simulink model "testbench_2"  (R2022b)
settings: Solver=VariableStepAuto  StartTime=0.0  StopTime=3600  RelTol=1e-3
undefined symbols (not defined in the file): battery_builder_rtmsupport, gcbh
libraries: nesl_utility x10, GD_Batterymodel_lib x8, fl_lib x2, BatteryCurrentManagement x1, BatteryBalancing x1
(part 1 of 2)
settings Model: Creator=DM  LastModifiedBy=DM

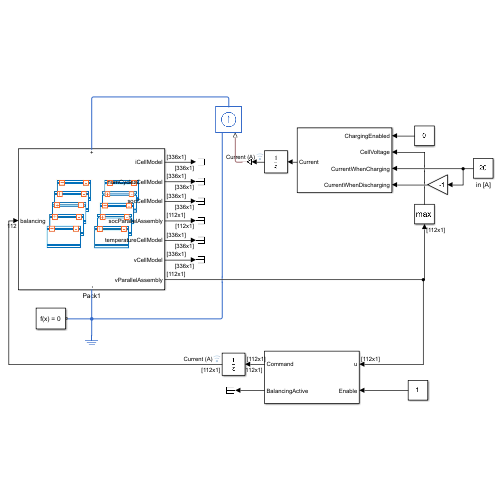
[thumbnail: Simulink's stored preview of the top-level diagram]
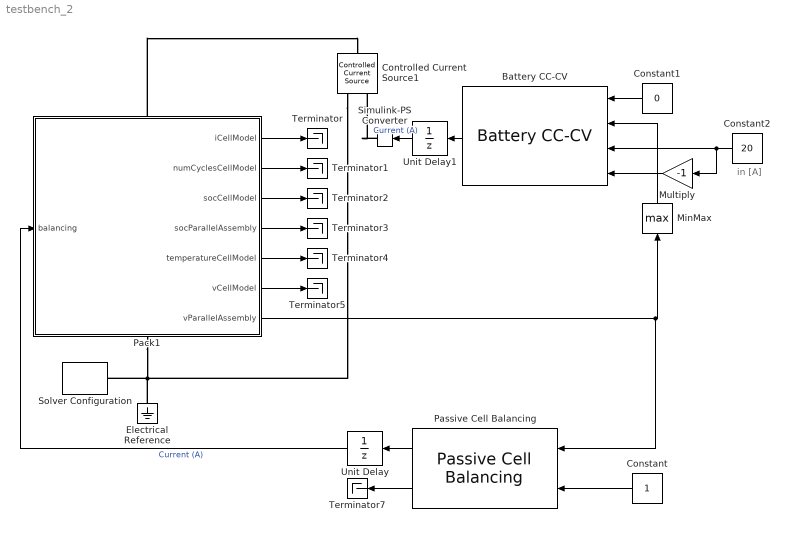
== system testbench_2 ==
  note: in [A]
  Battery CC-CV : BatteryCurrentManagement/Battery CC-CV  MaxCellVoltage=4.5  Kp=100  Ki=10  Kaw=1  Ts=-1
      settings: LibrarySourceBlock=batt_sl_lib/Current Management/Battery CC-CV
  Constant : Constant
  Constant1 : Constant  Value=0
  Constant2 : Constant  Value=20
  Controlled Current Source1 : fl_lib/Electrical/Electrical Sources/Controlled Current Source
  Electrical Reference : fl_lib/Electrical/Electrical Elements/Electrical Reference
  MinMax : MinMax  Function=max
  Multiply : Gain  Gain=-1
  Pack1 : Subsystem  LoadFcn=battery_builder_rtmsupport('loadfcn',gcbh);
      settings: CopyFcn=battery_builder_rtmsupport('copyfcn',gcbh);  PreCopyFcn=battery_builder_rtmsupport('precopyfcn',gcbh);  PreDeleteFcn=battery_builder_rtmsupport('predeletefcn',gcbh);  PortSchema="{\"entries\":[{\"content\":{\"sides\":[{\"content\":{\"connectorIds\":[\"LConn1\"]},\"type\":\"ConnectorPlacement.EquallySpacedRectSide\",\"uuid\":\"15f36c34-930d-4f52-9483-b00906672ad1\"},{\"content\":{\"connectorIds\":[\"RConn1\"],\"side\":\"RIGHT\"},\"type\":\"ConnectorPlacement.EquallySpacedRectSide\",\"uuid\":\"ac97c2df-2435-440c-95b5-222ce8189245\"},{\"content\":{\"connectorIds\":[\"In1\"],\"side\":\"TOP\"},\"type\":\"ConnectorPlacement.EquallySpacedRectSide\",\"uuid\":\"0c4398fe-7a4e-4114-b124-2a8e026b7d39\"},{\"content\":{\"connectorIds\":[\"Out1\",\"Out2\",\"Out3\",\"Out4\",\"Out5\",\"Out6\",\"Out7\"],\"side\":\"BOTTOM\"},\"type\":\"ConnectorPlacement.EquallySpacedRectSide\",\"uuid\":\"6740cf1b-9f23-4812-bda3-e18c05a0cb6c\"}]},\"type\":\"ConnectorPlacement.EquallySpacedConnector\",\"uuid\":\"12c02865-5fcb-4b07-b017-e8fa1f0f042b\"}],\"packageUris\":[\"http://schema.mathworks.com/mf0/Connector/R2020b\"],\"version\":\"1.0\"}"
      mask Display: image('$imagefile')
  Passive Cell Balancing : BatteryBalancing/Passive Cell Balancing  Threshold=0.2  Td_on=1  Td_off=1  Ts=-1
      settings: LibrarySourceBlock=batt_sl_lib/Cell Balancing/Passive Cell Balancing
  Simulink-PS Converter : nesl_utility/Simulink-PS Converter  PhysicalDomain=network_engine_domain  SubClassName=ps_input  LeftPortType=input  RightPortType=output  PseudoPeriodic=off  Frequencies=[]  NoiseDistribution=none  NoiseParameters=[]  Unit=1  AffineConversion=off  FilteringAndDerivatives=provide  SimscapeFilterOrder=1  InputFilterTimeConstant=0.001  UdotUserProvided=0
  Solver Configuration : nesl_utility/Solver Configuration  PhysicalDomain=network_engine_domain  SubClassName=solver  LeftPortType=input  RightPortType=generic  Tones=[]  Harmonics=[]  SimulateNoise=off  Profile=off  UseLocalSampling=off  EnableSwitchedLinearOptims=on  FrequencyDomain=off  UseCCode=off  RelTol=0.001  AbsTol=0.001  MinStep=1e-09  ToWorkspace=off  RevertToSquareIcSolve=off  NumHomotopyIterations=100  PhasorMode=off  PhasorModeNumHarmonics=1  ConsistencySolver=NEWTON_XTOL_AFTER_FTOL  IndexReductionMethod=DerivativeReplacement  DoDC=off  ResidualTolerance=1e-09  ConsistencyTolSource=GLOBAL  ConsistencyAbsTol=0.001  ConsistencyRelTol=0.001  ConsistencyTolFactor=0.001  UseLocalSolver=on  LocalSolverChoice=NE_BACKWARD_EULER_ADVANCER  ResolveIndetEquations=on  FunctionEvalNumThread=1  LocalSolverSampleTime=1  DoFixedCost=on  MaxNonlinIter=3  MaxModeIter=2  ComputeImpulses=off  ImpulseIterations=2  LinearAlgebra=auto  LinearAlgebraNumThread=0  EquationFormulation=NE_TIME_EF  DelaysMemoryBudget=1024  AutomaticFiltering=on  FilteringTimeConstant=0.001  PartitionStorageMethod=AS_NEEDED  PartitionMemoryBudget=1024  PartitionMethod=ROBUST
  Terminator{,1..5,7} (7 alike) : Terminator
  Unit Delay : UnitDelay  SampleTime=-1  HasFrameUpgradeWarning=on
  Unit Delay1 : UnitDelay  SampleTime=-1  HasFrameUpgradeWarning=on
  wires:
  Pack1/1(iCellModel) -> Terminator/1
  Pack1/2(numCyclesCellModel) -> Terminator1/1
  Pack1/3(socCellModel) -> Terminator2/1
  Pack1/4(socParallelAssembly) -> Terminator3/1
  Pack1/5(temperatureCellModel) -> Terminator4/1
  Pack1/6(vCellModel) -> Terminator5/1
  Passive Cell Balancing/2 -> Terminator7/1
  Constant/1 -> Passive Cell Balancing/2
  Constant1/1 -> Battery CC-CV/1
  Constant2/1 -> Multiply/1, Battery CC-CV/3
  Multiply/1 -> Battery CC-CV/4
  MinMax/1 -> Battery CC-CV/2
  Pack1/7(vParallelAssembly) -> Passive Cell Balancing/1, MinMax/1
  Passive Cell Balancing/1 -> Unit Delay/1
  Unit Delay/1 -> Pack1/1(balancing)  "Current (A)"
  Battery CC-CV/1 -> Unit Delay1/1
  Unit Delay1/1 -> Simulink-PS Converter/1  "Current (A)"
  connections:
  Pack1/LConn1 -- Controlled Current Source1/LConn1
  Electrical Reference/LConn1 -- Pack1/RConn1 -- Controlled Current Source1/RConn2 -- Solver Configuration/RConn1
  Simulink-PS Converter/RConn1 -- Controlled Current Source1/RConn1

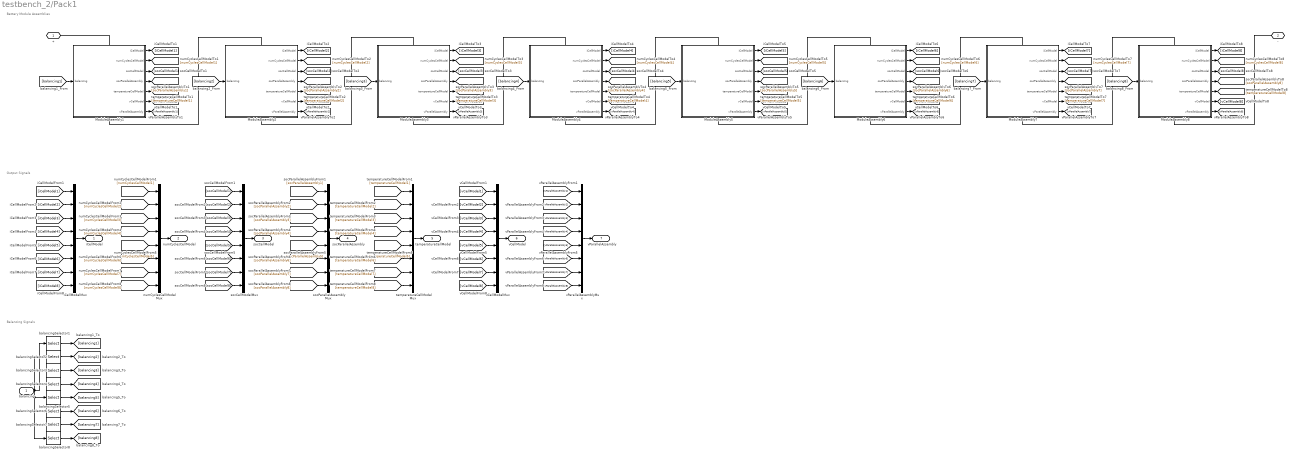
== system testbench_2/Pack1 ==
  note: Balancing Signals
  note: Output Signals
  note: Battery Module Assemblies
  balancing : Inport  PortDimensions=112
  ModuleAssembly1 : Subsystem  LoadFcn=battery_builder_rtmsupport('loadfcn',gcbh);
      settings: CopyFcn=battery_builder_rtmsupport('copyfcn',gcbh);  PreCopyFcn=battery_builder_rtmsupport('precopyfcn',gcbh);  PreDeleteFcn=battery_builder_rtmsupport('predeletefcn',gcbh);  PortSchema="{\"entries\":[{\"content\":{\"sides\":[{\"content\":{\"connectorIds\":[\"LConn1\"]},\"type\":\"ConnectorPlacement.EquallySpacedRectSide\",\"uuid\":\"15f36c34-930d-4f52-9483-b00906672ad1\"},{\"content\":{\"connectorIds\":[\"RConn1\"],\"side\":\"RIGHT\"},\"type\":\"ConnectorPlacement.EquallySpacedRectSide\",\"uuid\":\"ac97c2df-2435-440c-95b5-222ce8189245\"},{\"content\":{\"connectorIds\":[\"In1\"],\"side\":\"TOP\"},\"type\":\"ConnectorPlacement.EquallySpacedRectSide\",\"uuid\":\"0c4398fe-7a4e-4114-b124-2a8e026b7d39\"},{\"content\":{\"connectorIds\":[\"Out1\",\"Out2\",\"Out3\",\"Out4\",\"Out5\",\"Out6\",\"Out7\"],\"side\":\"BOTTOM\"},\"type\":\"ConnectorPlacement.EquallySpacedRectSide\",\"uuid\":\"5e29da8d-14fb-4ee5-a8e5-61c3c254e31c\"}]},\"type\":\"ConnectorPlacement.EquallySpacedConnector\",\"uuid\":\"12c02865-5fcb-4b07-b017-e8fa1f0f042b\"}],\"packageUris\":[\"http://schema.mathworks.com/mf0/Connector/R2020b\"],\"version\":\"1.0\"}"
      mask Display: image('$imagefile')
  ModuleAssembly2 : Subsystem  LoadFcn=battery_builder_rtmsupport('loadfcn',gcbh);
      settings: CopyFcn=battery_builder_rtmsupport('copyfcn',gcbh);  PreCopyFcn=battery_builder_rtmsupport('precopyfcn',gcbh);  PreDeleteFcn=battery_builder_rtmsupport('predeletefcn',gcbh);  PortSchema="{\"entries\":[{\"content\":{\"sides\":[{\"content\":{\"connectorIds\":[\"LConn1\"]},\"type\":\"ConnectorPlacement.EquallySpacedRectSide\",\"uuid\":\"15f36c34-930d-4f52-9483-b00906672ad1\"},{\"content\":{\"connectorIds\":[\"RConn1\"],\"side\":\"RIGHT\"},\"type\":\"ConnectorPlacement.EquallySpacedRectSide\",\"uuid\":\"ac97c2df-2435-440c-95b5-222ce8189245\"},{\"content\":{\"connectorIds\":[\"In1\"],\"side\":\"TOP\"},\"type\":\"ConnectorPlacement.EquallySpacedRectSide\",\"uuid\":\"0c4398fe-7a4e-4114-b124-2a8e026b7d39\"},{\"content\":{\"connectorIds\":[\"Out1\",\"Out2\",\"Out3\",\"Out4\",\"Out5\",\"Out6\",\"Out7\"],\"side\":\"BOTTOM\"},\"type\":\"ConnectorPlacement.EquallySpacedRectSide\",\"uuid\":\"5e29da8d-14fb-4ee5-a8e5-61c3c254e31c\"}]},\"type\":\"ConnectorPlacement.EquallySpacedConnector\",\"uuid\":\"12c02865-5fcb-4b07-b017-e8fa1f0f042b\"}],\"packageUris\":[\"http://schema.mathworks.com/mf0/Connector/R2020b\"],\"version\":\"1.0\"}"
      mask Display: image('$imagefile')
  ModuleAssembly3 : Subsystem  LoadFcn=battery_builder_rtmsupport('loadfcn',gcbh);
      settings: CopyFcn=battery_builder_rtmsupport('copyfcn',gcbh);  PreCopyFcn=battery_builder_rtmsupport('precopyfcn',gcbh);  PreDeleteFcn=battery_builder_rtmsupport('predeletefcn',gcbh);  PortSchema="{\"entries\":[{\"content\":{\"sides\":[{\"content\":{\"connectorIds\":[\"LConn1\"]},\"type\":\"ConnectorPlacement.EquallySpacedRectSide\",\"uuid\":\"15f36c34-930d-4f52-9483-b00906672ad1\"},{\"content\":{\"connectorIds\":[\"RConn1\"],\"side\":\"RIGHT\"},\"type\":\"ConnectorPlacement.EquallySpacedRectSide\",\"uuid\":\"ac97c2df-2435-440c-95b5-222ce8189245\"},{\"content\":{\"connectorIds\":[\"In1\"],\"side\":\"TOP\"},\"type\":\"ConnectorPlacement.EquallySpacedRectSide\",\"uuid\":\"0c4398fe-7a4e-4114-b124-2a8e026b7d39\"},{\"content\":{\"connectorIds\":[\"Out1\",\"Out2\",\"Out3\",\"Out4\",\"Out5\",\"Out6\",\"Out7\"],\"side\":\"BOTTOM\"},\"type\":\"ConnectorPlacement.EquallySpacedRectSide\",\"uuid\":\"5e29da8d-14fb-4ee5-a8e5-61c3c254e31c\"}]},\"type\":\"ConnectorPlacement.EquallySpacedConnector\",\"uuid\":\"12c02865-5fcb-4b07-b017-e8fa1f0f042b\"}],\"packageUris\":[\"http://schema.mathworks.com/mf0/Connector/R2020b\"],\"version\":\"1.0\"}"
      mask Display: image('$imagefile')
  ModuleAssembly4 : Subsystem  LoadFcn=battery_builder_rtmsupport('loadfcn',gcbh);
      settings: CopyFcn=battery_builder_rtmsupport('copyfcn',gcbh);  PreCopyFcn=battery_builder_rtmsupport('precopyfcn',gcbh);  PreDeleteFcn=battery_builder_rtmsupport('predeletefcn',gcbh);  PortSchema="{\"entries\":[{\"content\":{\"sides\":[{\"content\":{\"connectorIds\":[\"LConn1\"]},\"type\":\"ConnectorPlacement.EquallySpacedRectSide\",\"uuid\":\"15f36c34-930d-4f52-9483-b00906672ad1\"},{\"content\":{\"connectorIds\":[\"RConn1\"],\"side\":\"RIGHT\"},\"type\":\"ConnectorPlacement.EquallySpacedRectSide\",\"uuid\":\"ac97c2df-2435-440c-95b5-222ce8189245\"},{\"content\":{\"connectorIds\":[\"In1\"],\"side\":\"TOP\"},\"type\":\"ConnectorPlacement.EquallySpacedRectSide\",\"uuid\":\"0c4398fe-7a4e-4114-b124-2a8e026b7d39\"},{\"content\":{\"connectorIds\":[\"Out1\",\"Out2\",\"Out3\",\"Out4\",\"Out5\",\"Out6\",\"Out7\"],\"side\":\"BOTTOM\"},\"type\":\"ConnectorPlacement.EquallySpacedRectSide\",\"uuid\":\"5e29da8d-14fb-4ee5-a8e5-61c3c254e31c\"}]},\"type\":\"ConnectorPlacement.EquallySpacedConnector\",\"uuid\":\"12c02865-5fcb-4b07-b017-e8fa1f0f042b\"}],\"packageUris\":[\"http://schema.mathworks.com/mf0/Connector/R2020b\"],\"version\":\"1.0\"}"
      mask Display: image('$imagefile')
  ModuleAssembly5 : Subsystem  LoadFcn=battery_builder_rtmsupport('loadfcn',gcbh);
      settings: CopyFcn=battery_builder_rtmsupport('copyfcn',gcbh);  PreCopyFcn=battery_builder_rtmsupport('precopyfcn',gcbh);  PreDeleteFcn=battery_builder_rtmsupport('predeletefcn',gcbh);  PortSchema="{\"entries\":[{\"content\":{\"sides\":[{\"content\":{\"connectorIds\":[\"LConn1\"]},\"type\":\"ConnectorPlacement.EquallySpacedRectSide\",\"uuid\":\"15f36c34-930d-4f52-9483-b00906672ad1\"},{\"content\":{\"connectorIds\":[\"RConn1\"],\"side\":\"RIGHT\"},\"type\":\"ConnectorPlacement.EquallySpacedRectSide\",\"uuid\":\"ac97c2df-2435-440c-95b5-222ce8189245\"},{\"content\":{\"connectorIds\":[\"In1\"],\"side\":\"TOP\"},\"type\":\"ConnectorPlacement.EquallySpacedRectSide\",\"uuid\":\"0c4398fe-7a4e-4114-b124-2a8e026b7d39\"},{\"content\":{\"connectorIds\":[\"Out1\",\"Out2\",\"Out3\",\"Out4\",\"Out5\",\"Out6\",\"Out7\"],\"side\":\"BOTTOM\"},\"type\":\"ConnectorPlacement.EquallySpacedRectSide\",\"uuid\":\"5e29da8d-14fb-4ee5-a8e5-61c3c254e31c\"}]},\"type\":\"ConnectorPlacement.EquallySpacedConnector\",\"uuid\":\"12c02865-5fcb-4b07-b017-e8fa1f0f042b\"}],\"packageUris\":[\"http://schema.mathworks.com/mf0/Connector/R2020b\"],\"version\":\"1.0\"}"
      mask Display: image('$imagefile')
  ModuleAssembly6 : Subsystem  LoadFcn=battery_builder_rtmsupport('loadfcn',gcbh);
      settings: CopyFcn=battery_builder_rtmsupport('copyfcn',gcbh);  PreCopyFcn=battery_builder_rtmsupport('precopyfcn',gcbh);  PreDeleteFcn=battery_builder_rtmsupport('predeletefcn',gcbh);  PortSchema="{\"entries\":[{\"content\":{\"sides\":[{\"content\":{\"connectorIds\":[\"LConn1\"]},\"type\":\"ConnectorPlacement.EquallySpacedRectSide\",\"uuid\":\"15f36c34-930d-4f52-9483-b00906672ad1\"},{\"content\":{\"connectorIds\":[\"RConn1\"],\"side\":\"RIGHT\"},\"type\":\"ConnectorPlacement.EquallySpacedRectSide\",\"uuid\":\"ac97c2df-2435-440c-95b5-222ce8189245\"},{\"content\":{\"connectorIds\":[\"In1\"],\"side\":\"TOP\"},\"type\":\"ConnectorPlacement.EquallySpacedRectSide\",\"uuid\":\"0c4398fe-7a4e-4114-b124-2a8e026b7d39\"},{\"content\":{\"connectorIds\":[\"Out1\",\"Out2\",\"Out3\",\"Out4\",\"Out5\",\"Out6\",\"Out7\"],\"side\":\"BOTTOM\"},\"type\":\"ConnectorPlacement.EquallySpacedRectSide\",\"uuid\":\"5e29da8d-14fb-4ee5-a8e5-61c3c254e31c\"}]},\"type\":\"ConnectorPlacement.EquallySpacedConnector\",\"uuid\":\"12c02865-5fcb-4b07-b017-e8fa1f0f042b\"}],\"packageUris\":[\"http://schema.mathworks.com/mf0/Connector/R2020b\"],\"version\":\"1.0\"}"
      mask Display: image('$imagefile')
  ModuleAssembly7 : Subsystem  LoadFcn=battery_builder_rtmsupport('loadfcn',gcbh);
      settings: CopyFcn=battery_builder_rtmsupport('copyfcn',gcbh);  PreCopyFcn=battery_builder_rtmsupport('precopyfcn',gcbh);  PreDeleteFcn=battery_builder_rtmsupport('predeletefcn',gcbh);  PortSchema="{\"entries\":[{\"content\":{\"sides\":[{\"content\":{\"connectorIds\":[\"LConn1\"]},\"type\":\"ConnectorPlacement.EquallySpacedRectSide\",\"uuid\":\"15f36c34-930d-4f52-9483-b00906672ad1\"},{\"content\":{\"connectorIds\":[\"RConn1\"],\"side\":\"RIGHT\"},\"type\":\"ConnectorPlacement.EquallySpacedRectSide\",\"uuid\":\"ac97c2df-2435-440c-95b5-222ce8189245\"},{\"content\":{\"connectorIds\":[\"In1\"],\"side\":\"TOP\"},\"type\":\"ConnectorPlacement.EquallySpacedRectSide\",\"uuid\":\"0c4398fe-7a4e-4114-b124-2a8e026b7d39\"},{\"content\":{\"connectorIds\":[\"Out1\",\"Out2\",\"Out3\",\"Out4\",\"Out5\",\"Out6\",\"Out7\"],\"side\":\"BOTTOM\"},\"type\":\"ConnectorPlacement.EquallySpacedRectSide\",\"uuid\":\"5e29da8d-14fb-4ee5-a8e5-61c3c254e31c\"}]},\"type\":\"ConnectorPlacement.EquallySpacedConnector\",\"uuid\":\"12c02865-5fcb-4b07-b017-e8fa1f0f042b\"}],\"packageUris\":[\"http://schema.mathworks.com/mf0/Connector/R2020b\"],\"version\":\"1.0\"}"
      mask Display: image('$imagefile')
  ModuleAssembly8 : Subsystem  LoadFcn=battery_builder_rtmsupport('loadfcn',gcbh);
      settings: CopyFcn=battery_builder_rtmsupport('copyfcn',gcbh);  PreCopyFcn=battery_builder_rtmsupport('precopyfcn',gcbh);  PreDeleteFcn=battery_builder_rtmsupport('predeletefcn',gcbh);  PortSchema="{\"entries\":[{\"content\":{\"sides\":[{\"content\":{\"connectorIds\":[\"LConn1\"]},\"type\":\"ConnectorPlacement.EquallySpacedRectSide\",\"uuid\":\"15f36c34-930d-4f52-9483-b00906672ad1\"},{\"content\":{\"connectorIds\":[\"RConn1\"],\"side\":\"RIGHT\"},\"type\":\"ConnectorPlacement.EquallySpacedRectSide\",\"uuid\":\"ac97c2df-2435-440c-95b5-222ce8189245\"},{\"content\":{\"connectorIds\":[\"In1\"],\"side\":\"TOP\"},\"type\":\"ConnectorPlacement.EquallySpacedRectSide\",\"uuid\":\"0c4398fe-7a4e-4114-b124-2a8e026b7d39\"},{\"content\":{\"connectorIds\":[\"Out1\",\"Out2\",\"Out3\",\"Out4\",\"Out5\",\"Out6\",\"Out7\"],\"side\":\"BOTTOM\"},\"type\":\"ConnectorPlacement.EquallySpacedRectSide\",\"uuid\":\"5e29da8d-14fb-4ee5-a8e5-61c3c254e31c\"}]},\"type\":\"ConnectorPlacement.EquallySpacedConnector\",\"uuid\":\"12c02865-5fcb-4b07-b017-e8fa1f0f042b\"}],\"packageUris\":[\"http://schema.mathworks.com/mf0/Connector/R2020b\"],\"version\":\"1.0\"}"
      mask Display: image('$imagefile')
  balancingSelector1 : Selector  InputPortWidth=112  IndexOptions=Index vector (dialog)  Indices="[1   2   3   4   5   6   7   8   9  10  11  12  13  14]"  OutputSizes=1
  balancingSelector2 : Selector  InputPortWidth=112  IndexOptions=Index vector (dialog)  Indices="[15  16  17  18  19  20  21  22  23  24  25  26  27  28]"  OutputSizes=1
  balancingSelector3 : Selector  InputPortWidth=112  IndexOptions=Index vector (dialog)  Indices="[29  30  31  32  33  34  35  36  37  38  39  40  41  42]"  OutputSizes=1
  balancingSelector4 : Selector  InputPortWidth=112  IndexOptions=Index vector (dialog)  Indices="[43  44  45  46  47  48  49  50  51  52  53  54  55  56]"  OutputSizes=1
  balancingSelector5 : Selector  InputPortWidth=112  IndexOptions=Index vector (dialog)  Indices="[57  58  59  60  61  62  63  64  65  66  67  68  69  70]"  OutputSizes=1
  balancingSelector6 : Selector  InputPortWidth=112  IndexOptions=Index vector (dialog)  Indices="[71  72  73  74  75  76  77  78  79  80  81  82  83  84]"  OutputSizes=1
  balancingSelector7 : Selector  InputPortWidth=112  IndexOptions=Index vector (dialog)  Indices="[85  86  87  88  89  90  91  92  93  94  95  96  97  98]"  OutputSizes=1
  balancingSelector8 : Selector  InputPortWidth=112  IndexOptions=Index vector (dialog)  Indices="[99  100  101  102  103  104  105  106  107  108  109  110  111  112]"  OutputSizes=1
  iCellModelMux : Mux  Inputs=8
  numCyclesCellModelMux : Mux  Inputs=8
  socCellModelMux : Mux  Inputs=8
  socParallelAssemblyMux : Mux  Inputs=8
  temperatureCellModelMux : Mux  Inputs=8
  vCellModelMux : Mux  Inputs=8
  vParallelAssemblyMux : Mux  Inputs=8
  + : PMIOPort  Side=Left
  - : PMIOPort  Port=2  Side=Right
  iCellModel : Outport
  numCyclesCellModel : Outport  Port=2
  socCellModel : Outport  Port=3
  socParallelAssembly : Outport  Port=4
  temperatureCellModel : Outport  Port=5
  vCellModel : Outport  Port=6
  vParallelAssembly : Outport  Port=7
  wires:
  [balancing8] -> ModuleAssembly8/1(balancing)
  balancingSelector8/1 -> [balancing8]
  [balancing7] -> ModuleAssembly7/1(balancing)
  balancingSelector7/1 -> [balancing7]
  [balancing6] -> ModuleAssembly6/1(balancing)
  balancingSelector6/1 -> [balancing6]
  [balancing5] -> ModuleAssembly5/1(balancing)
  balancingSelector5/1 -> [balancing5]
  [balancing4] -> ModuleAssembly4/1(balancing)
  balancingSelector4/1 -> [balancing4]
  [balancing3] -> ModuleAssembly3/1(balancing)
  balancingSelector3/1 -> [balancing3]
  [balancing2] -> ModuleAssembly2/1(balancing)
  balancingSelector2/1 -> [balancing2]
  [balancing1] -> ModuleAssembly1/1(balancing)
  balancing/1 -> balancingSelector1/1, balancingSelector4/1, balancingSelector3/1, balancingSelector2/1, balancingSelector5/1, balancingSelector6/1, balancingSelector8/1, balancingSelector7/1
  balancingSelector1/1 -> [balancing1]
  [vParallelAssembly8] -> vParallelAssemblyMux/8
  ModuleAssembly8/7(vParallelAssembly) -> [vParallelAssembly8]
  [vCellModel8] -> vCellModelMux/8
  ModuleAssembly8/6(vCellModel) -> [vCellModel8]
  [temperatureCellModel8] -> temperatureCellModelMux/8
  ModuleAssembly8/5(temperatureCellModel) -> [temperatureCellModel8]
  [socParallelAssembly8] -> socParallelAssemblyMux/8
  ModuleAssembly8/4(socParallelAssembly) -> [socParallelAssembly8]
  [socCellModel8] -> socCellModelMux/8
  ModuleAssembly8/3(socCellModel) -> [socCellModel8]
  [numCyclesCellModel8] -> numCyclesCellModelMux/8
  ModuleAssembly8/2(numCyclesCellModel) -> [numCyclesCellModel8]
  [iCellModel8] -> iCellModelMux/8
  ModuleAssembly8/1(iCellModel) -> [iCellModel8]
  [vParallelAssembly7] -> vParallelAssemblyMux/7
  ModuleAssembly7/7(vParallelAssembly) -> [vParallelAssembly7]
  [vCellModel7] -> vCellModelMux/7
  ModuleAssembly7/6(vCellModel) -> [vCellModel7]
  [temperatureCellModel7] -> temperatureCellModelMux/7
  ModuleAssembly7/5(temperatureCellModel) -> [temperatureCellModel7]
  [socParallelAssembly7] -> socParallelAssemblyMux/7
  ModuleAssembly7/4(socParallelAssembly) -> [socParallelAssembly7]
  [socCellModel7] -> socCellModelMux/7
  ModuleAssembly7/3(socCellModel) -> [socCellModel7]
  [numCyclesCellModel7] -> numCyclesCellModelMux/7
  ModuleAssembly7/2(numCyclesCellModel) -> [numCyclesCellModel7]
  [iCellModel7] -> iCellModelMux/7
  ModuleAssembly7/1(iCellModel) -> [iCellModel7]
  [vParallelAssembly6] -> vParallelAssemblyMux/6
  ModuleAssembly6/7(vParallelAssembly) -> [vParallelAssembly6]
  [vCellModel6] -> vCellModelMux/6
  ModuleAssembly6/6(vCellModel) -> [vCellModel6]
  [temperatureCellModel6] -> temperatureCellModelMux/6
  ModuleAssembly6/5(temperatureCellModel) -> [temperatureCellModel6]
  [socParallelAssembly6] -> socParallelAssemblyMux/6
  ModuleAssembly6/4(socParallelAssembly) -> [socParallelAssembly6]
  [socCellModel6] -> socCellModelMux/6
  ModuleAssembly6/3(socCellModel) -> [socCellModel6]
  [numCyclesCellModel6] -> numCyclesCellModelMux/6
  ModuleAssembly6/2(numCyclesCellModel) -> [numCyclesCellModel6]
  [iCellModel6] -> iCellModelMux/6
  ModuleAssembly6/1(iCellModel) -> [iCellModel6]
  [vParallelAssembly5] -> vParallelAssemblyMux/5
  ModuleAssembly5/7(vParallelAssembly) -> [vParallelAssembly5]
  [vCellModel5] -> vCellModelMux/5
  ModuleAssembly5/6(vCellModel) -> [vCellModel5]
  [temperatureCellModel5] -> temperatureCellModelMux/5
  ModuleAssembly5/5(temperatureCellModel) -> [temperatureCellModel5]
  [socParallelAssembly5] -> socParallelAssemblyMux/5
  ModuleAssembly5/4(socParallelAssembly) -> [socParallelAssembly5]
  [socCellModel5] -> socCellModelMux/5
  ModuleAssembly5/3(socCellModel) -> [socCellModel5]
  [numCyclesCellModel5] -> numCyclesCellModelMux/5
  ModuleAssembly5/2(numCyclesCellModel) -> [numCyclesCellModel5]
  [iCellModel5] -> iCellModelMux/5
  ModuleAssembly5/1(iCellModel) -> [iCellModel5]
  [vParallelAssembly4] -> vParallelAssemblyMux/4
  ModuleAssembly4/7(vParallelAssembly) -> [vParallelAssembly4]
  [vCellModel4] -> vCellModelMux/4
  ModuleAssembly4/6(vCellModel) -> [vCellModel4]
  [temperatureCellModel4] -> temperatureCellModelMux/4
  ModuleAssembly4/5(temperatureCellModel) -> [temperatureCellModel4]
  [socParallelAssembly4] -> socParallelAssemblyMux/4
  ModuleAssembly4/4(socParallelAssembly) -> [socParallelAssembly4]
  [socCellModel4] -> socCellModelMux/4
  ModuleAssembly4/3(socCellModel) -> [socCellModel4]
  [numCyclesCellModel4] -> numCyclesCellModelMux/4
  ModuleAssembly4/2(numCyclesCellModel) -> [numCyclesCellModel4]
  [iCellModel4] -> iCellModelMux/4
  ModuleAssembly4/1(iCellModel) -> [iCellModel4]
  [vParallelAssembly3] -> vParallelAssemblyMux/3
  ModuleAssembly3/7(vParallelAssembly) -> [vParallelAssembly3]
  [vCellModel3] -> vCellModelMux/3
  ModuleAssembly3/6(vCellModel) -> [vCellModel3]
  [temperatureCellModel3] -> temperatureCellModelMux/3
  ModuleAssembly3/5(temperatureCellModel) -> [temperatureCellModel3]
  [socParallelAssembly3] -> socParallelAssemblyMux/3
  ModuleAssembly3/4(socParallelAssembly) -> [socParallelAssembly3]
  [socCellModel3] -> socCellModelMux/3
  ModuleAssembly3/3(socCellModel) -> [socCellModel3]
  [numCyclesCellModel3] -> numCyclesCellModelMux/3
  ModuleAssembly3/2(numCyclesCellModel) -> [numCyclesCellModel3]
  [iCellModel3] -> iCellModelMux/3
  ModuleAssembly3/1(iCellModel) -> [iCellModel3]
  [vParallelAssembly2] -> vParallelAssemblyMux/2
  ModuleAssembly2/7(vParallelAssembly) -> [vParallelAssembly2]
  [vCellModel2] -> vCellModelMux/2
  ModuleAssembly2/6(vCellModel) -> [vCellModel2]
  [temperatureCellModel2] -> temperatureCellModelMux/2
  ModuleAssembly2/5(temperatureCellModel) -> [temperatureCellModel2]
  [socParallelAssembly2] -> socParallelAssemblyMux/2
  ModuleAssembly2/4(socParallelAssembly) -> [socParallelAssembly2]
  [socCellModel2] -> socCellModelMux/2
  ModuleAssembly2/3(socCellModel) -> [socCellModel2]
  [numCyclesCellModel2] -> numCyclesCellModelMux/2
  ModuleAssembly2/2(numCyclesCellModel) -> [numCyclesCellModel2]
  [iCellModel2] -> iCellModelMux/2
  ModuleAssembly2/1(iCellModel) -> [iCellModel2]
  [vParallelAssembly1] -> vParallelAssemblyMux/1
  vParallelAssemblyMux/1 -> vParallelAssembly/1
  ModuleAssembly1/7(vParallelAssembly) -> [vParallelAssembly1]
  [vCellModel1] -> vCellModelMux/1
  vCellModelMux/1 -> vCellModel/1
  ModuleAssembly1/6(vCellModel) -> [vCellModel1]
  [temperatureCellModel1] -> temperatureCellModelMux/1
  temperatureCellModelMux/1 -> temperatureCellModel/1
  ModuleAssembly1/5(temperatureCellModel) -> [temperatureCellModel1]
  [socParallelAssembly1] -> socParallelAssemblyMux/1
  socParallelAssemblyMux/1 -> socParallelAssembly/1
  ModuleAssembly1/4(socParallelAssembly) -> [socParallelAssembly1]
  [socCellModel1] -> socCellModelMux/1
  socCellModelMux/1 -> socCellModel/1
  ModuleAssembly1/3(socCellModel) -> [socCellModel1]
  [numCyclesCellModel1] -> numCyclesCellModelMux/1
  numCyclesCellModelMux/1 -> numCyclesCellModel/1
  ModuleAssembly1/2(numCyclesCellModel) -> [numCyclesCellModel1]
  [iCellModel1] -> iCellModelMux/1
  iCellModelMux/1 -> iCellModel/1
  ModuleAssembly1/1(iCellModel) -> [iCellModel1]
  connections:
  ModuleAssembly8/RConn1 -- -/RConn1
  ModuleAssembly1/LConn1 -- +/RConn1
  ModuleAssembly8/LConn1 -- ModuleAssembly7/RConn1
  ModuleAssembly7/LConn1 -- ModuleAssembly6/RConn1
  ModuleAssembly6/LConn1 -- ModuleAssembly5/RConn1
  ModuleAssembly5/LConn1 -- ModuleAssembly4/RConn1
  ModuleAssembly4/LConn1 -- ModuleAssembly3/RConn1
  ModuleAssembly3/LConn1 -- ModuleAssembly2/RConn1
  ModuleAssembly2/LConn1 -- ModuleAssembly1/RConn1

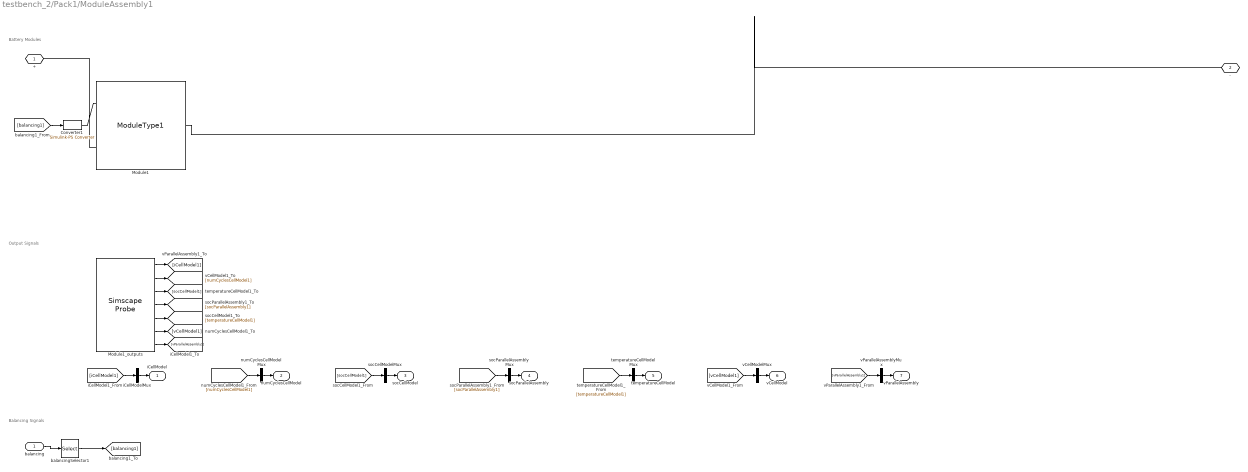
== system testbench_2/Pack1/ModuleAssembly1 ==
  note: Battery Modules
  note: Output Signals
  note: Balancing Signals
  balancing : Inport  PortDimensions=14
  Converter1 : nesl_utility/Simulink-PS Converter  PhysicalDomain=network_engine_domain  SubClassName=ps_input  LeftPortType=input  RightPortType=output  PseudoPeriodic=off  Frequencies=[]  NoiseDistribution=none  NoiseParameters=[]  Unit=1  AffineConversion=off  FilteringAndDerivatives=provide  SimscapeFilterOrder=1  InputFilterTimeConstant=0.001  UdotUserProvided=0
  Module1 : GD_Batterymodel_lib/Modules/ModuleType1  SOC_vec=[0, .1, .25, .5, .75, .9, 1]  T_vec=[278, 293, 313] K  V0_mat=[3.49, 3.5, 3.51; 3.55, 3.57, 3.56; 3.62, 3.63, 3.64; 3.71, 3.71, 3.72; 3.91, 3.93, 3.94; 4.07, 4.08, 4.08; 4.19, 4.19, 4.19] V  V_range=[0, inf] V  R0_mat=[.0117, .0085, .009; .011, .0085, .009; .0114, .0087, .0092; .0107, .0082, .0088; .0107, .0083, .0091; .0113, .0085, .0089; .0116, .0085, .0089] Ohm  AH=27 A*hr  extrapolation_option=simscape.enum.extrapolation.nearest  thermal_mass=100 J/K  CellBalancingClosedResistance=0.01 Ohm  CellBalancingOpenConductance=1e-8 1/Ohm  CellBalancingThreshold=0.5  CellBalancingResistance=50 Ohm  P=3  S=14  iCellModel_specify=off  iCellModel_priority=None  iCellModel=repmat(0, 42, 1) A  iCellModel_nominal_specify=off  iCellModel_nominal_unit=A  iCellModel_nominal_value=1  vCellModel_specify=off  vCellModel_priority=None  vCellModel=repmat(0, 42, 1) V  vCellModel_nominal_specify=off  vCellModel_nominal_unit=V  vCellModel_nominal_value=1  socCellModel_specify=off  socCellModel_priority=High  socCellModel=repmat(1, 42, 1)  socCellModel_nominal_specify=off  socCellModel_nominal_unit=1  socCellModel_nominal_value=1  numCyclesCellModel_specify=off  numCyclesCellModel_priority=High  numCyclesCellModel=repmat(0, 42, 1)  numCyclesCellModel_nominal_specify=off  numCyclesCellModel_nominal_unit=1  numCyclesCellModel_nominal_value=1  temperatureCellModel_specify=off  temperatureCellModel_priority=High  temperatureCellModel=repmat(298.15, 42, 1) K  temperatureCellModel_nominal_specify=off  temperatureCellModel_nominal_unit=K  temperatureCellModel_nominal_value=1  vParallelAssembly_specify=off  vParallelAssembly_priority=None  vParallelAssembly=repmat(0, 14, 1) V  vParallelAssembly_nominal_specify=off  vParallelAssembly_nominal_unit=V  vParallelAssembly_nominal_value=1  socParallelAssembly_specify=off  socParallelAssembly_priority=None  socParallelAssembly=repmat(1, 14, 1)  socParallelAssembly_nominal_specify=off  socParallelAssembly_nominal_unit=1  socParallelAssembly_nominal_value=1
      settings: InternalSimscapePortConfiguration="{\"Bottom\":[{\"id\":\"n\",\"label\":\"-\",\"type\":\"foundation.electrical.electrical\"}],\"Left\":[{\"id\":\"enableCellBalancing\",\"label\":\"CB\",\"type\":\"input\"}],\"Right\":[],\"Top\":[{\"id\":\"p\",\"label\":\"+\",\"type\":\"foundation.electrical.electrical\"}]}"
  Module1_outputs : SimscapeProbe  BoundBlock=522  Variables={iCellModel, numCyclesCellModel, socCellModel, socParallelAssembly, temperatureCellModel, vCellModel, vParallelAssembly}
  balancingSelector1 : Selector  InputPortWidth=14  IndexOptions=Index vector (dialog)  Indices="[1   2   3   4   5   6   7   8   9  10  11  12  13  14]"  OutputSizes=1
  iCellModelMux : Mux  Inputs=1
  numCyclesCellModelMux : Mux  Inputs=1
  socCellModelMux : Mux  Inputs=1
  socParallelAssemblyMux : Mux  Inputs=1
  temperatureCellModelMux : Mux  Inputs=1
  vCellModelMux : Mux  Inputs=1
  vParallelAssemblyMux : Mux  Inputs=1
  + : PMIOPort  Side=Left
  - : PMIOPort  Port=2  Side=Right
  iCellModel : Outport
  numCyclesCellModel : Outport  Port=2
  socCellModel : Outport  Port=3
  socParallelAssembly : Outport  Port=4
  temperatureCellModel : Outport  Port=5
  vCellModel : Outport  Port=6
  vParallelAssembly : Outport  Port=7
  wires:
  Module1_outputs/7 -> [vParallelAssembly1]
  iCellModelMux/1 -> iCellModel/1
  [iCellModel1] -> iCellModelMux/1
  Module1_outputs/6 -> [vCellModel1]
  numCyclesCellModelMux/1 -> numCyclesCellModel/1
  [numCyclesCellModel1] -> numCyclesCellModelMux/1
  Module1_outputs/5 -> [temperatureCellModel1]
  socCellModelMux/1 -> socCellModel/1
  [socCellModel1] -> socCellModelMux/1
  Module1_outputs/4 -> [socParallelAssembly1]
  socParallelAssemblyMux/1 -> socParallelAssembly/1
  [socParallelAssembly1] -> socParallelAssemblyMux/1
  Module1_outputs/3 -> [socCellModel1]
  temperatureCellModelMux/1 -> temperatureCellModel/1
  [temperatureCellModel1] -> temperatureCellModelMux/1
  Module1_outputs/2 -> [numCyclesCellModel1]
  vCellModelMux/1 -> vCellModel/1
  [vCellModel1] -> vCellModelMux/1
  Module1_outputs/1 -> [iCellModel1]
  vParallelAssemblyMux/1 -> vParallelAssembly/1
  [vParallelAssembly1] -> vParallelAssemblyMux/1
  balancing/1 -> balancingSelector1/1
  balancingSelector1/1 -> [balancing1]
  [balancing1] -> Converter1/1
  connections:
  Module1/LConn2 -- +/RConn1
  Module1/RConn1 -- -/RConn1
  Converter1/RConn1 -- Module1/LConn1

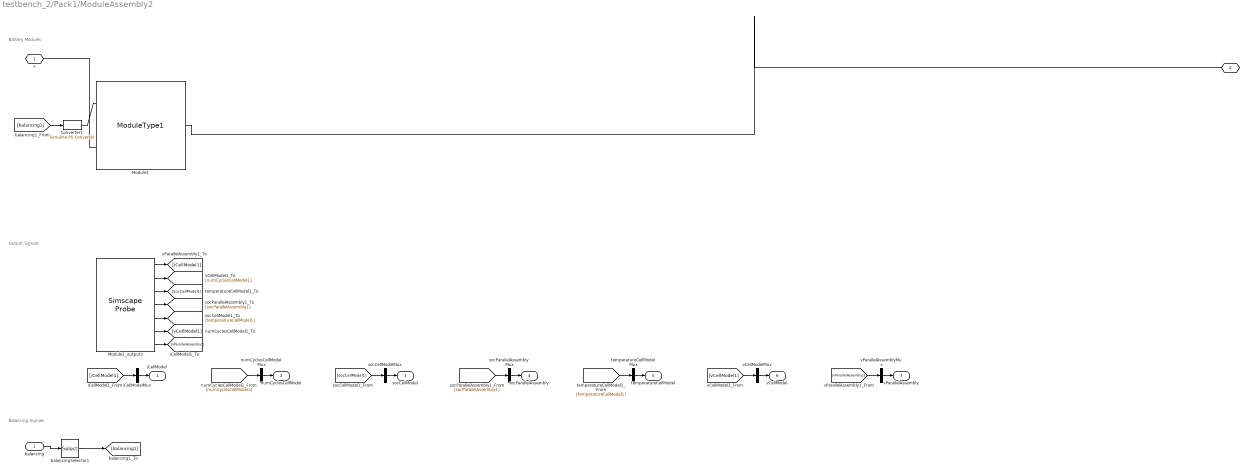
== system testbench_2/Pack1/ModuleAssembly2 ==
  note: Battery Modules
  note: Output Signals
  note: Balancing Signals
  balancing : Inport  PortDimensions=14
  Converter1 : nesl_utility/Simulink-PS Converter  PhysicalDomain=network_engine_domain  SubClassName=ps_input  LeftPortType=input  RightPortType=output  PseudoPeriodic=off  Frequencies=[]  NoiseDistribution=none  NoiseParameters=[]  Unit=1  AffineConversion=off  FilteringAndDerivatives=provide  SimscapeFilterOrder=1  InputFilterTimeConstant=0.001  UdotUserProvided=0
  Module1 : GD_Batterymodel_lib/Modules/ModuleType1  SOC_vec=[0, .1, .25, .5, .75, .9, 1]  T_vec=[278, 293, 313] K  V0_mat=[3.49, 3.5, 3.51; 3.55, 3.57, 3.56; 3.62, 3.63, 3.64; 3.71, 3.71, 3.72; 3.91, 3.93, 3.94; 4.07, 4.08, 4.08; 4.19, 4.19, 4.19] V  V_range=[0, inf] V  R0_mat=[.0117, .0085, .009; .011, .0085, .009; .0114, .0087, .0092; .0107, .0082, .0088; .0107, .0083, .0091; .0113, .0085, .0089; .0116, .0085, .0089] Ohm  AH=27 A*hr  extrapolation_option=simscape.enum.extrapolation.nearest  thermal_mass=100 J/K  CellBalancingClosedResistance=0.01 Ohm  CellBalancingOpenConductance=1e-8 1/Ohm  CellBalancingThreshold=0.5  CellBalancingResistance=50 Ohm  P=3  S=14  iCellModel_specify=off  iCellModel_priority=None  iCellModel=repmat(0, 42, 1) A  iCellModel_nominal_specify=off  iCellModel_nominal_unit=A  iCellModel_nominal_value=1  vCellModel_specify=off  vCellModel_priority=None  vCellModel=repmat(0, 42, 1) V  vCellModel_nominal_specify=off  vCellModel_nominal_unit=V  vCellModel_nominal_value=1  socCellModel_specify=off  socCellModel_priority=High  socCellModel=repmat(1, 42, 1)  socCellModel_nominal_specify=off  socCellModel_nominal_unit=1  socCellModel_nominal_value=1  numCyclesCellModel_specify=off  numCyclesCellModel_priority=High  numCyclesCellModel=repmat(0, 42, 1)  numCyclesCellModel_nominal_specify=off  numCyclesCellModel_nominal_unit=1  numCyclesCellModel_nominal_value=1  temperatureCellModel_specify=off  temperatureCellModel_priority=High  temperatureCellModel=repmat(298.15, 42, 1) K  temperatureCellModel_nominal_specify=off  temperatureCellModel_nominal_unit=K  temperatureCellModel_nominal_value=1  vParallelAssembly_specify=off  vParallelAssembly_priority=None  vParallelAssembly=repmat(0, 14, 1) V  vParallelAssembly_nominal_specify=off  vParallelAssembly_nominal_unit=V  vParallelAssembly_nominal_value=1  socParallelAssembly_specify=off  socParallelAssembly_priority=None  socParallelAssembly=repmat(1, 14, 1)  socParallelAssembly_nominal_specify=off  socParallelAssembly_nominal_unit=1  socParallelAssembly_nominal_value=1
      settings: InternalSimscapePortConfiguration="{\"Bottom\":[{\"id\":\"n\",\"label\":\"-\",\"type\":\"foundation.electrical.electrical\"}],\"Left\":[{\"id\":\"enableCellBalancing\",\"label\":\"CB\",\"type\":\"input\"}],\"Right\":[],\"Top\":[{\"id\":\"p\",\"label\":\"+\",\"type\":\"foundation.electrical.electrical\"}]}"
  Module1_outputs : SimscapeProbe  BoundBlock=563  Variables={iCellModel, numCyclesCellModel, socCellModel, socParallelAssembly, temperatureCellModel, vCellModel, vParallelAssembly}
  balancingSelector1 : Selector  InputPortWidth=14  IndexOptions=Index vector (dialog)  Indices="[1   2   3   4   5   6   7   8   9  10  11  12  13  14]"  OutputSizes=1
  iCellModelMux : Mux  Inputs=1
  numCyclesCellModelMux : Mux  Inputs=1
  socCellModelMux : Mux  Inputs=1
  socParallelAssemblyMux : Mux  Inputs=1
  temperatureCellModelMux : Mux  Inputs=1
  vCellModelMux : Mux  Inputs=1
  vParallelAssemblyMux : Mux  Inputs=1
  + : PMIOPort  Side=Left
  - : PMIOPort  Port=2  Side=Right
  iCellModel : Outport
  numCyclesCellModel : Outport  Port=2
  socCellModel : Outport  Port=3
  socParallelAssembly : Outport  Port=4
  temperatureCellModel : Outport  Port=5
  vCellModel : Outport  Port=6
  vParallelAssembly : Outport  Port=7
  wires:
  Module1_outputs/7 -> [vParallelAssembly1]
  iCellModelMux/1 -> iCellModel/1
  [iCellModel1] -> iCellModelMux/1
  Module1_outputs/6 -> [vCellModel1]
  numCyclesCellModelMux/1 -> numCyclesCellModel/1
  [numCyclesCellModel1] -> numCyclesCellModelMux/1
  Module1_outputs/5 -> [temperatureCellModel1]
  socCellModelMux/1 -> socCellModel/1
  [socCellModel1] -> socCellModelMux/1
  Module1_outputs/4 -> [socParallelAssembly1]
  socParallelAssemblyMux/1 -> socParallelAssembly/1
  [socParallelAssembly1] -> socParallelAssemblyMux/1
  Module1_outputs/3 -> [socCellModel1]
  temperatureCellModelMux/1 -> temperatureCellModel/1
  [temperatureCellModel1] -> temperatureCellModelMux/1
  Module1_outputs/2 -> [numCyclesCellModel1]
  vCellModelMux/1 -> vCellModel/1
  [vCellModel1] -> vCellModelMux/1
  Module1_outputs/1 -> [iCellModel1]
  vParallelAssemblyMux/1 -> vParallelAssembly/1
  [vParallelAssembly1] -> vParallelAssemblyMux/1
  balancing/1 -> balancingSelector1/1
  balancingSelector1/1 -> [balancing1]
  [balancing1] -> Converter1/1
  connections:
  Module1/LConn2 -- +/RConn1
  Module1/RConn1 -- -/RConn1
  Converter1/RConn1 -- Module1/LConn1

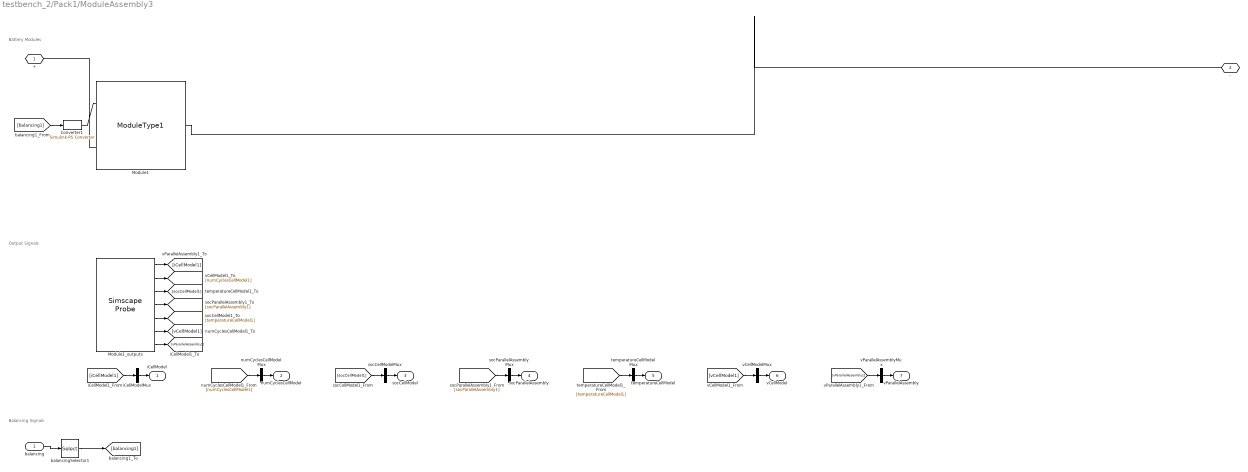
== system testbench_2/Pack1/ModuleAssembly3 ==
  note: Battery Modules
  note: Output Signals
  note: Balancing Signals
  balancing : Inport  PortDimensions=14
  Converter1 : nesl_utility/Simulink-PS Converter  PhysicalDomain=network_engine_domain  SubClassName=ps_input  LeftPortType=input  RightPortType=output  PseudoPeriodic=off  Frequencies=[]  NoiseDistribution=none  NoiseParameters=[]  Unit=1  AffineConversion=off  FilteringAndDerivatives=provide  SimscapeFilterOrder=1  InputFilterTimeConstant=0.001  UdotUserProvided=0
  Module1 : GD_Batterymodel_lib/Modules/ModuleType1  SOC_vec=[0, .1, .25, .5, .75, .9, 1]  T_vec=[278, 293, 313] K  V0_mat=[3.49, 3.5, 3.51; 3.55, 3.57, 3.56; 3.62, 3.63, 3.64; 3.71, 3.71, 3.72; 3.91, 3.93, 3.94; 4.07, 4.08, 4.08; 4.19, 4.19, 4.19] V  V_range=[0, inf] V  R0_mat=[.0117, .0085, .009; .011, .0085, .009; .0114, .0087, .0092; .0107, .0082, .0088; .0107, .0083, .0091; .0113, .0085, .0089; .0116, .0085, .0089] Ohm  AH=27 A*hr  extrapolation_option=simscape.enum.extrapolation.nearest  thermal_mass=100 J/K  CellBalancingClosedResistance=0.01 Ohm  CellBalancingOpenConductance=1e-8 1/Ohm  CellBalancingThreshold=0.5  CellBalancingResistance=50 Ohm  P=3  S=14  iCellModel_specify=off  iCellModel_priority=None  iCellModel=repmat(0, 42, 1) A  iCellModel_nominal_specify=off  iCellModel_nominal_unit=A  iCellModel_nominal_value=1  vCellModel_specify=off  vCellModel_priority=None  vCellModel=repmat(0, 42, 1) V  vCellModel_nominal_specify=off  vCellModel_nominal_unit=V  vCellModel_nominal_value=1  socCellModel_specify=off  socCellModel_priority=High  socCellModel=repmat(1, 42, 1)  socCellModel_nominal_specify=off  socCellModel_nominal_unit=1  socCellModel_nominal_value=1  numCyclesCellModel_specify=off  numCyclesCellModel_priority=High  numCyclesCellModel=repmat(0, 42, 1)  numCyclesCellModel_nominal_specify=off  numCyclesCellModel_nominal_unit=1  numCyclesCellModel_nominal_value=1  temperatureCellModel_specify=off  temperatureCellModel_priority=High  temperatureCellModel=repmat(298.15, 42, 1) K  temperatureCellModel_nominal_specify=off  temperatureCellModel_nominal_unit=K  temperatureCellModel_nominal_value=1  vParallelAssembly_specify=off  vParallelAssembly_priority=None  vParallelAssembly=repmat(0, 14, 1) V  vParallelAssembly_nominal_specify=off  vParallelAssembly_nominal_unit=V  vParallelAssembly_nominal_value=1  socParallelAssembly_specify=off  socParallelAssembly_priority=None  socParallelAssembly=repmat(1, 14, 1)  socParallelAssembly_nominal_specify=off  socParallelAssembly_nominal_unit=1  socParallelAssembly_nominal_value=1
      settings: InternalSimscapePortConfiguration="{\"Bottom\":[{\"id\":\"n\",\"label\":\"-\",\"type\":\"foundation.electrical.electrical\"}],\"Left\":[{\"id\":\"enableCellBalancing\",\"label\":\"CB\",\"type\":\"input\"}],\"Right\":[],\"Top\":[{\"id\":\"p\",\"label\":\"+\",\"type\":\"foundation.electrical.electrical\"}]}"
  Module1_outputs : SimscapeProbe  BoundBlock=604  Variables={iCellModel, numCyclesCellModel, socCellModel, socParallelAssembly, temperatureCellModel, vCellModel, vParallelAssembly}
  balancingSelector1 : Selector  InputPortWidth=14  IndexOptions=Index vector (dialog)  Indices="[1   2   3   4   5   6   7   8   9  10  11  12  13  14]"  OutputSizes=1
  iCellModelMux : Mux  Inputs=1
  numCyclesCellModelMux : Mux  Inputs=1
  socCellModelMux : Mux  Inputs=1
  socParallelAssemblyMux : Mux  Inputs=1
  temperatureCellModelMux : Mux  Inputs=1
  vCellModelMux : Mux  Inputs=1
  vParallelAssemblyMux : Mux  Inputs=1
  + : PMIOPort  Side=Left
  - : PMIOPort  Port=2  Side=Right
  iCellModel : Outport
  numCyclesCellModel : Outport  Port=2
  socCellModel : Outport  Port=3
  socParallelAssembly : Outport  Port=4
  temperatureCellModel : Outport  Port=5
  vCellModel : Outport  Port=6
  vParallelAssembly : Outport  Port=7
  wires:
  Module1_outputs/7 -> [vParallelAssembly1]
  iCellModelMux/1 -> iCellModel/1
  [iCellModel1] -> iCellModelMux/1
  Module1_outputs/6 -> [vCellModel1]
  numCyclesCellModelMux/1 -> numCyclesCellModel/1
  [numCyclesCellModel1] -> numCyclesCellModelMux/1
  Module1_outputs/5 -> [temperatureCellModel1]
  socCellModelMux/1 -> socCellModel/1
  [socCellModel1] -> socCellModelMux/1
  Module1_outputs/4 -> [socParallelAssembly1]
  socParallelAssemblyMux/1 -> socParallelAssembly/1
  [socParallelAssembly1] -> socParallelAssemblyMux/1
  Module1_outputs/3 -> [socCellModel1]
  temperatureCellModelMux/1 -> temperatureCellModel/1
  [temperatureCellModel1] -> temperatureCellModelMux/1
  Module1_outputs/2 -> [numCyclesCellModel1]
  vCellModelMux/1 -> vCellModel/1
  [vCellModel1] -> vCellModelMux/1
  Module1_outputs/1 -> [iCellModel1]
  vParallelAssemblyMux/1 -> vParallelAssembly/1
  [vParallelAssembly1] -> vParallelAssemblyMux/1
  balancing/1 -> balancingSelector1/1
  balancingSelector1/1 -> [balancing1]
  [balancing1] -> Converter1/1
  connections:
  Module1/LConn2 -- +/RConn1
  Module1/RConn1 -- -/RConn1
  Converter1/RConn1 -- Module1/LConn1

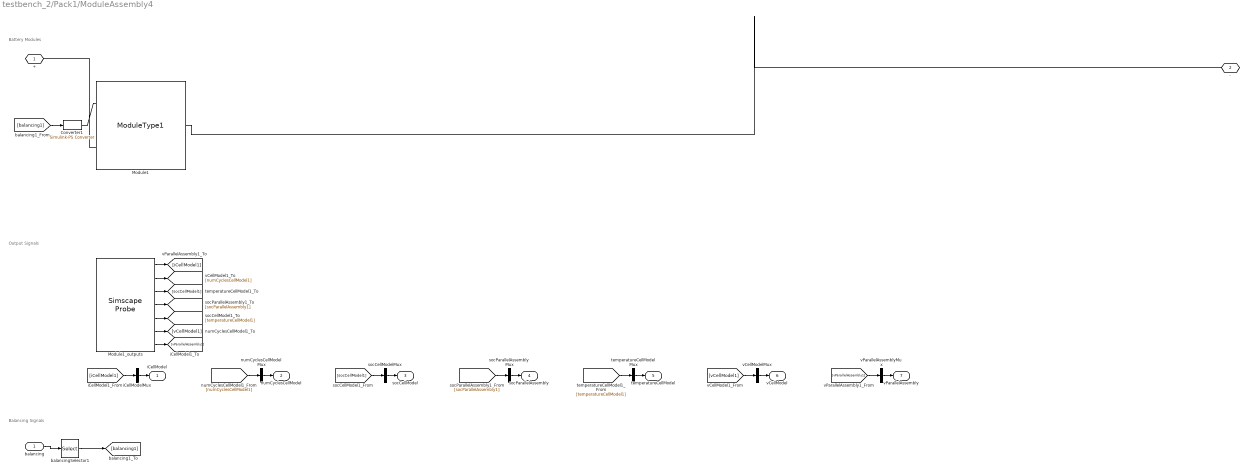
== system testbench_2/Pack1/ModuleAssembly4 ==
  note: Battery Modules
  note: Output Signals
  note: Balancing Signals
  balancing : Inport  PortDimensions=14
  Converter1 : nesl_utility/Simulink-PS Converter  PhysicalDomain=network_engine_domain  SubClassName=ps_input  LeftPortType=input  RightPortType=output  PseudoPeriodic=off  Frequencies=[]  NoiseDistribution=none  NoiseParameters=[]  Unit=1  AffineConversion=off  FilteringAndDerivatives=provide  SimscapeFilterOrder=1  InputFilterTimeConstant=0.001  UdotUserProvided=0
  Module1 : GD_Batterymodel_lib/Modules/ModuleType1  SOC_vec=[0, .1, .25, .5, .75, .9, 1]  T_vec=[278, 293, 313] K  V0_mat=[3.49, 3.5, 3.51; 3.55, 3.57, 3.56; 3.62, 3.63, 3.64; 3.71, 3.71, 3.72; 3.91, 3.93, 3.94; 4.07, 4.08, 4.08; 4.19, 4.19, 4.19] V  V_range=[0, inf] V  R0_mat=[.0117, .0085, .009; .011, .0085, .009; .0114, .0087, .0092; .0107, .0082, .0088; .0107, .0083, .0091; .0113, .0085, .0089; .0116, .0085, .0089] Ohm  AH=27 A*hr  extrapolation_option=simscape.enum.extrapolation.nearest  thermal_mass=100 J/K  CellBalancingClosedResistance=0.01 Ohm  CellBalancingOpenConductance=1e-8 1/Ohm  CellBalancingThreshold=0.5  CellBalancingResistance=50 Ohm  P=3  S=14  iCellModel_specify=off  iCellModel_priority=None  iCellModel=repmat(0, 42, 1) A  iCellModel_nominal_specify=off  iCellModel_nominal_unit=A  iCellModel_nominal_value=1  vCellModel_specify=off  vCellModel_priority=None  vCellModel=repmat(0, 42, 1) V  vCellModel_nominal_specify=off  vCellModel_nominal_unit=V  vCellModel_nominal_value=1  socCellModel_specify=off  socCellModel_priority=High  socCellModel=repmat(1, 42, 1)  socCellModel_nominal_specify=off  socCellModel_nominal_unit=1  socCellModel_nominal_value=1  numCyclesCellModel_specify=off  numCyclesCellModel_priority=High  numCyclesCellModel=repmat(0, 42, 1)  numCyclesCellModel_nominal_specify=off  numCyclesCellModel_nominal_unit=1  numCyclesCellModel_nominal_value=1  temperatureCellModel_specify=off  temperatureCellModel_priority=High  temperatureCellModel=repmat(298.15, 42, 1) K  temperatureCellModel_nominal_specify=off  temperatureCellModel_nominal_unit=K  temperatureCellModel_nominal_value=1  vParallelAssembly_specify=off  vParallelAssembly_priority=None  vParallelAssembly=repmat(0, 14, 1) V  vParallelAssembly_nominal_specify=off  vParallelAssembly_nominal_unit=V  vParallelAssembly_nominal_value=1  socParallelAssembly_specify=off  socParallelAssembly_priority=None  socParallelAssembly=repmat(1, 14, 1)  socParallelAssembly_nominal_specify=off  socParallelAssembly_nominal_unit=1  socParallelAssembly_nominal_value=1
      settings: InternalSimscapePortConfiguration="{\"Bottom\":[{\"id\":\"n\",\"label\":\"-\",\"type\":\"foundation.electrical.electrical\"}],\"Left\":[{\"id\":\"enableCellBalancing\",\"label\":\"CB\",\"type\":\"input\"}],\"Right\":[],\"Top\":[{\"id\":\"p\",\"label\":\"+\",\"type\":\"foundation.electrical.electrical\"}]}"
  Module1_outputs : SimscapeProbe  BoundBlock=645  Variables={iCellModel, numCyclesCellModel, socCellModel, socParallelAssembly, temperatureCellModel, vCellModel, vParallelAssembly}
  balancingSelector1 : Selector  InputPortWidth=14  IndexOptions=Index vector (dialog)  Indices="[1   2   3   4   5   6   7   8   9  10  11  12  13  14]"  OutputSizes=1
  iCellModelMux : Mux  Inputs=1
  numCyclesCellModelMux : Mux  Inputs=1
  socCellModelMux : Mux  Inputs=1
  socParallelAssemblyMux : Mux  Inputs=1
  temperatureCellModelMux : Mux  Inputs=1
  vCellModelMux : Mux  Inputs=1
  vParallelAssemblyMux : Mux  Inputs=1
  + : PMIOPort  Side=Left
  - : PMIOPort  Port=2  Side=Right
  iCellModel : Outport
  numCyclesCellModel : Outport  Port=2
  socCellModel : Outport  Port=3
  socParallelAssembly : Outport  Port=4
  temperatureCellModel : Outport  Port=5
  vCellModel : Outport  Port=6
  vParallelAssembly : Outport  Port=7
  wires:
  Module1_outputs/7 -> [vParallelAssembly1]
  iCellModelMux/1 -> iCellModel/1
  [iCellModel1] -> iCellModelMux/1
  Module1_outputs/6 -> [vCellModel1]
  numCyclesCellModelMux/1 -> numCyclesCellModel/1
  [numCyclesCellModel1] -> numCyclesCellModelMux/1
  Module1_outputs/5 -> [temperatureCellModel1]
  socCellModelMux/1 -> socCellModel/1
  [socCellModel1] -> socCellModelMux/1
  Module1_outputs/4 -> [socParallelAssembly1]
  socParallelAssemblyMux/1 -> socParallelAssembly/1
  [socParallelAssembly1] -> socParallelAssemblyMux/1
  Module1_outputs/3 -> [socCellModel1]
  temperatureCellModelMux/1 -> temperatureCellModel/1
  [temperatureCellModel1] -> temperatureCellModelMux/1
  Module1_outputs/2 -> [numCyclesCellModel1]
  vCellModelMux/1 -> vCellModel/1
  [vCellModel1] -> vCellModelMux/1
  Module1_outputs/1 -> [iCellModel1]
  vParallelAssemblyMux/1 -> vParallelAssembly/1
  [vParallelAssembly1] -> vParallelAssemblyMux/1
  balancing/1 -> balancingSelector1/1
  balancingSelector1/1 -> [balancing1]
  [balancing1] -> Converter1/1
  connections:
  Module1/LConn2 -- +/RConn1
  Module1/RConn1 -- -/RConn1
  Converter1/RConn1 -- Module1/LConn1

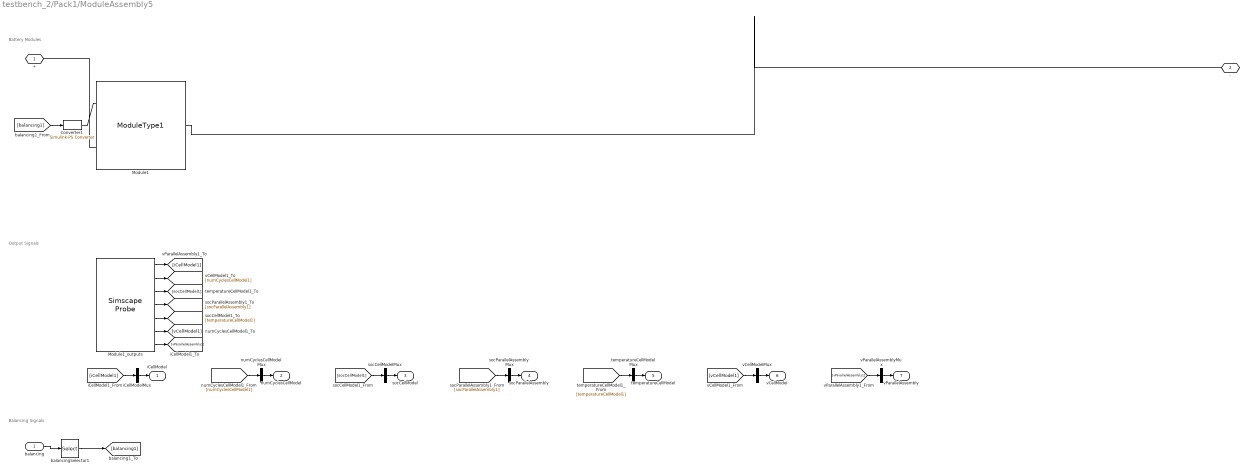
== system testbench_2/Pack1/ModuleAssembly5 ==
  note: Battery Modules
  note: Output Signals
  note: Balancing Signals
  balancing : Inport  PortDimensions=14
  Converter1 : nesl_utility/Simulink-PS Converter  PhysicalDomain=network_engine_domain  SubClassName=ps_input  LeftPortType=input  RightPortType=output  PseudoPeriodic=off  Frequencies=[]  NoiseDistribution=none  NoiseParameters=[]  Unit=1  AffineConversion=off  FilteringAndDerivatives=provide  SimscapeFilterOrder=1  InputFilterTimeConstant=0.001  UdotUserProvided=0
  Module1 : GD_Batterymodel_lib/Modules/ModuleType1  SOC_vec=[0, .1, .25, .5, .75, .9, 1]  T_vec=[278, 293, 313] K  V0_mat=[3.49, 3.5, 3.51; 3.55, 3.57, 3.56; 3.62, 3.63, 3.64; 3.71, 3.71, 3.72; 3.91, 3.93, 3.94; 4.07, 4.08, 4.08; 4.19, 4.19, 4.19] V  V_range=[0, inf] V  R0_mat=[.0117, .0085, .009; .011, .0085, .009; .0114, .0087, .0092; .0107, .0082, .0088; .0107, .0083, .0091; .0113, .0085, .0089; .0116, .0085, .0089] Ohm  AH=27 A*hr  extrapolation_option=simscape.enum.extrapolation.nearest  thermal_mass=100 J/K  CellBalancingClosedResistance=0.01 Ohm  CellBalancingOpenConductance=1e-8 1/Ohm  CellBalancingThreshold=0.5  CellBalancingResistance=50 Ohm  P=3  S=14  iCellModel_specify=off  iCellModel_priority=None  iCellModel=repmat(0, 42, 1) A  iCellModel_nominal_specify=off  iCellModel_nominal_unit=A  iCellModel_nominal_value=1  vCellModel_specify=off  vCellModel_priority=None  vCellModel=repmat(0, 42, 1) V  vCellModel_nominal_specify=off  vCellModel_nominal_unit=V  vCellModel_nominal_value=1  socCellModel_specify=off  socCellModel_priority=High  socCellModel=repmat(1, 42, 1)  socCellModel_nominal_specify=off  socCellModel_nominal_unit=1  socCellModel_nominal_value=1  numCyclesCellModel_specify=off  numCyclesCellModel_priority=High  numCyclesCellModel=repmat(0, 42, 1)  numCyclesCellModel_nominal_specify=off  numCyclesCellModel_nominal_unit=1  numCyclesCellModel_nominal_value=1  temperatureCellModel_specify=off  temperatureCellModel_priority=High  temperatureCellModel=repmat(298.15, 42, 1) K  temperatureCellModel_nominal_specify=off  temperatureCellModel_nominal_unit=K  temperatureCellModel_nominal_value=1  vParallelAssembly_specify=off  vParallelAssembly_priority=None  vParallelAssembly=repmat(0, 14, 1) V  vParallelAssembly_nominal_specify=off  vParallelAssembly_nominal_unit=V  vParallelAssembly_nominal_value=1  socParallelAssembly_specify=off  socParallelAssembly_priority=None  socParallelAssembly=repmat(1, 14, 1)  socParallelAssembly_nominal_specify=off  socParallelAssembly_nominal_unit=1  socParallelAssembly_nominal_value=1
      settings: InternalSimscapePortConfiguration="{\"Bottom\":[{\"id\":\"n\",\"label\":\"-\",\"type\":\"foundation.electrical.electrical\"}],\"Left\":[{\"id\":\"enableCellBalancing\",\"label\":\"CB\",\"type\":\"input\"}],\"Right\":[],\"Top\":[{\"id\":\"p\",\"label\":\"+\",\"type\":\"foundation.electrical.electrical\"}]}"
  Module1_outputs : SimscapeProbe  BoundBlock=686  Variables={iCellModel, numCyclesCellModel, socCellModel, socParallelAssembly, temperatureCellModel, vCellModel, vParallelAssembly}
  balancingSelector1 : Selector  InputPortWidth=14  IndexOptions=Index vector (dialog)  Indices="[1   2   3   4   5   6   7   8   9  10  11  12  13  14]"  OutputSizes=1
  iCellModelMux : Mux  Inputs=1
  numCyclesCellModelMux : Mux  Inputs=1
  socCellModelMux : Mux  Inputs=1
  socParallelAssemblyMux : Mux  Inputs=1
  temperatureCellModelMux : Mux  Inputs=1
  vCellModelMux : Mux  Inputs=1
  vParallelAssemblyMux : Mux  Inputs=1
  + : PMIOPort  Side=Left
  - : PMIOPort  Port=2  Side=Right
  iCellModel : Outport
  numCyclesCellModel : Outport  Port=2
  socCellModel : Outport  Port=3
  socParallelAssembly : Outport  Port=4
  temperatureCellModel : Outport  Port=5
  vCellModel : Outport  Port=6
  vParallelAssembly : Outport  Port=7
  wires:
  Module1_outputs/7 -> [vParallelAssembly1]
  iCellModelMux/1 -> iCellModel/1
  [iCellModel1] -> iCellModelMux/1
  Module1_outputs/6 -> [vCellModel1]
  numCyclesCellModelMux/1 -> numCyclesCellModel/1
  [numCyclesCellModel1] -> numCyclesCellModelMux/1
  Module1_outputs/5 -> [temperatureCellModel1]
  socCellModelMux/1 -> socCellModel/1
  [socCellModel1] -> socCellModelMux/1
  Module1_outputs/4 -> [socParallelAssembly1]
  socParallelAssemblyMux/1 -> socParallelAssembly/1
  [socParallelAssembly1] -> socParallelAssemblyMux/1
  Module1_outputs/3 -> [socCellModel1]
  temperatureCellModelMux/1 -> temperatureCellModel/1
  [temperatureCellModel1] -> temperatureCellModelMux/1
  Module1_outputs/2 -> [numCyclesCellModel1]
  vCellModelMux/1 -> vCellModel/1
  [vCellModel1] -> vCellModelMux/1
  Module1_outputs/1 -> [iCellModel1]
  vParallelAssemblyMux/1 -> vParallelAssembly/1
  [vParallelAssembly1] -> vParallelAssemblyMux/1
  balancing/1 -> balancingSelector1/1
  balancingSelector1/1 -> [balancing1]
  [balancing1] -> Converter1/1
  connections:
  Module1/LConn2 -- +/RConn1
  Module1/RConn1 -- -/RConn1
  Converter1/RConn1 -- Module1/LConn1
